simulink model "admittance_controller_sim_hardware"  (R2023b)
settings: Solver=FixedStepAuto  StartTime=0.0  StopTime=inf  RelTol=1e-3  EnableMultiTasking=on
values from neighbouring files (symbols this model uses):
  A_discr = c2d(A,0.005,'Tustin')    [admittance_controller.m]
undefined symbols (not defined in the file or in its folder): DiscIntNeverNeededParam, K, Ts
libraries: simulink_extras x2
settings Model: ExtModeTrigDuration=10  Creator=paoli  LastModifiedBy=kiraa
settings OptimizationCC: EnhancedBackFolding=on  PassReuseOutputArgsAs=Individual arguments  ZeroExternalMemoryAtStartup=off  ZeroInternalMemoryAtStartup=off  MaxStackSize=64  OptimizeBlockOrder=speed  DifferentSizesBufferReuse=on  OptimizationCustomize=off  EfficientTunableParamExpr=on
settings DebuggingCC: ParameterTunabilityLossMsg=error
settings HardwareCC: ProdBitPerPointer=32  ProdBitPerSizeT=32  ProdBitPerPtrDiffT=32  ProdLargestAtomicInteger=Long  ProdLargestAtomicFloat=Double  ProdWordSize=32  ProdLongLongMode=on  ProdHWDeviceType=ARM Compatible->ARM Cortex
settings SFSimCC: MATLABDynamicMemAlloc=off
settings RTWCC: Description=Embedded Coder  SystemTargetFile=ert.tlc  HardwareBoard=STM32 Nucleo F401RE  TemplateMakefile=ert_default_tmf  Toolchain=GNU Tools for ARM Embedded Processors
settings CodeAppCC: ForceParamTrailComments=on  IgnoreCustomStorageClasses=off  OperatorAnnotations=on  SimulinkDataObjDesc=on  SFDataObjDesc=on  InsertBlockDesc=on
settings ERTTargetCC: SupportContinuousTime=on  ExtModeTransport=3  ExtModeStaticAlloc=on  ExtModeStaticAllocSize=2000  ExtModeMexFile=ext_xcp  ExtModeIntrfLevel=Level2 - Open

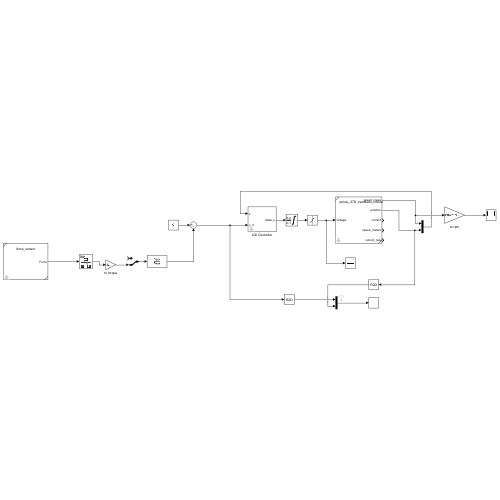
[thumbnail: Simulink's stored preview of the top-level diagram]
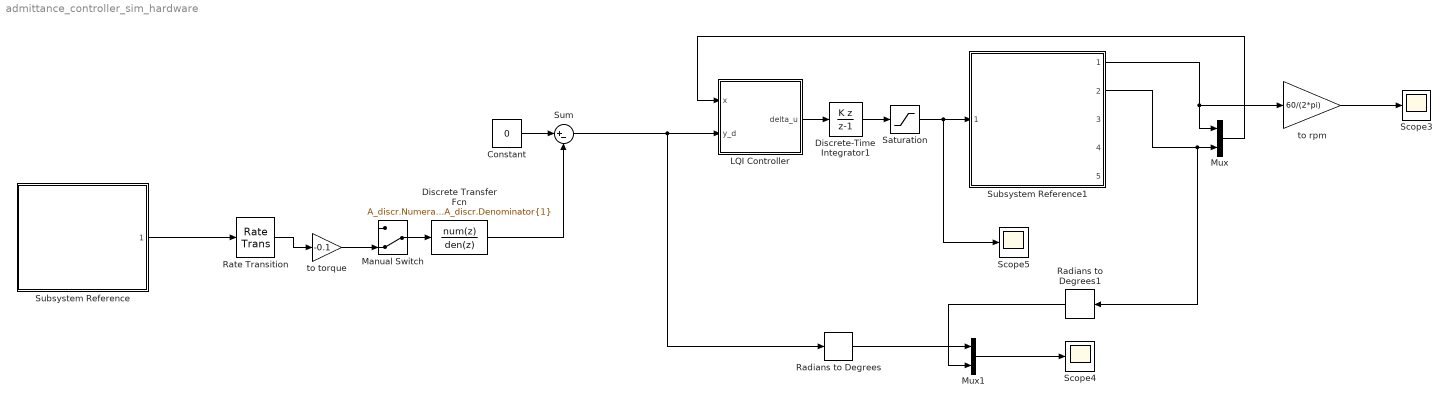
== system admittance_controller_sim_hardware ==
  Constant : Constant  Value=0
  Discrete Transfer Fcn : DiscreteTransferFcn  Numerator=A_discr.Numerator{1}  Denominator=A_discr.Denominator{1}  SampleTime=0.005
  Discrete-Time Integrator1 : DiscreteIntegrator  IntegratorMethod=Accumulation: Backward Euler  SampleTime=Ts  LimitOutput=on  UpperSaturationLimit=12  LowerSaturationLimit=-12  ICPrevOutput=DiscIntNeverNeededParam  ICPrevScaledInput=DiscIntNeverNeededParam
  LQI Controller : Subsystem  mask{Ts=0.005}
  Manual Switch : ManualSwitch  CurrentSetting=0
  Mux : Mux  Inputs=2
  Mux1 : Mux  Inputs=2
  Radians to Degrees : simulink_extras/Transformations/Radians to Degrees
  Radians to Degrees1 : simulink_extras/Transformations/Radians to Degrees
  Rate Transition : RateTransition
  Saturation : Saturate  UpperLimit=12  LowerLimit=-12
  Scope3 : Scope
  Scope4 : Scope
  Scope5 : Scope
  Subsystem Reference : Subsystem  ReferencedSubsystem=force_sensor  Ts=0.001
  Subsystem Reference1 : Subsystem  ReferencedSubsystem=pololu_37D_hardware_interface  Ts=0.005  pwmFreq=2000
  Sum : Sum  Inputs=|+-
  to rpm : Gain  Gain=60/(2*pi)
  to torque : Gain  Gain=-0.1
  wires:
  Mux/1 -> LQI Controller/1(x)
  Subsystem Reference1/1 -> Mux/1, to rpm/1
  Subsystem Reference1/2 -> Radians to Degrees1/1, Mux/2
  to rpm/1 -> Scope3/1
  Mux1/1 -> Scope4/1
  Radians to Degrees/1 -> Mux1/1
  Radians to Degrees1/1 -> Mux1/2
  Saturation/1 -> Subsystem Reference1/1, Scope5/1
  LQI Controller/1(delta_u) -> Discrete-Time Integrator1/1
  Discrete-Time Integrator1/1 -> Saturation/1
  Sum/1 -> Radians to Degrees/1, LQI Controller/2(y_d)
  Constant/1 -> Sum/1
  Discrete Transfer Fcn/1 -> Sum/2
  Manual Switch/1 -> Discrete Transfer Fcn/1
  to torque/1 -> Manual Switch/2
  Subsystem Reference/1 -> Rate Transition/1
  Rate Transition/1 -> to torque/1

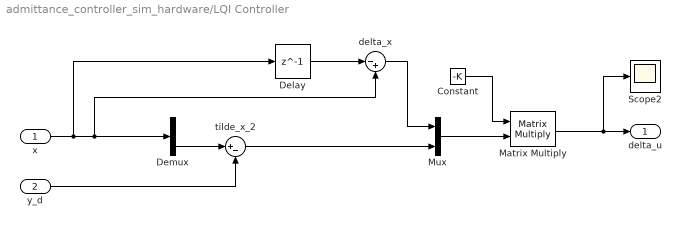
== system admittance_controller_sim_hardware/LQI Controller ==
  x : Inport  SampleTime=Ts
  y_d : Inport  Port=2  SampleTime=Ts
  Constant : Constant  Value=-K  VectorParams1D=off
  Delay : Delay  DelayLength=1  InitialCondition=[0;0]  SampleTime=Ts
  Demux : Demux  Outputs=2
  Matrix Multiply : Product  Multiplication=Matrix(*)
  Mux : Mux  Inputs=2
  Scope2 : Scope
  delta_x : Sum  Inputs=|-+
  tilde_x_2 : Sum  Inputs=|+-
  delta_u : Outport  SampleTime=Ts
  wires:
  x/1 -> Delay/1, delta_x/2, Demux/1
  Mux/1 -> Matrix Multiply/2
  Demux/2 -> tilde_x_2/1
  y_d/1 -> tilde_x_2/2
  Delay/1 -> delta_x/1
  tilde_x_2/1 -> Mux/2
  Matrix Multiply/1 -> Scope2/1, delta_u/1
  Constant/1 -> Matrix Multiply/1
  delta_x/1 -> Mux/1
